simulink model "nonlinear_block"  (R2024b)
settings: Solver=ode45  StartTime=0.0  StopTime=20  FixedStep=0.01  RelTol=1e-4  AbsTol=1e-7
undefined symbols (not defined in the file): params
settings Model: Creator=david  LastModifiedBy=david

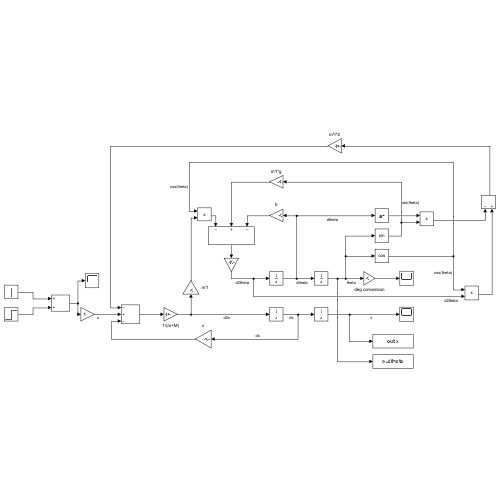
[thumbnail: Simulink's stored preview of the top-level diagram]
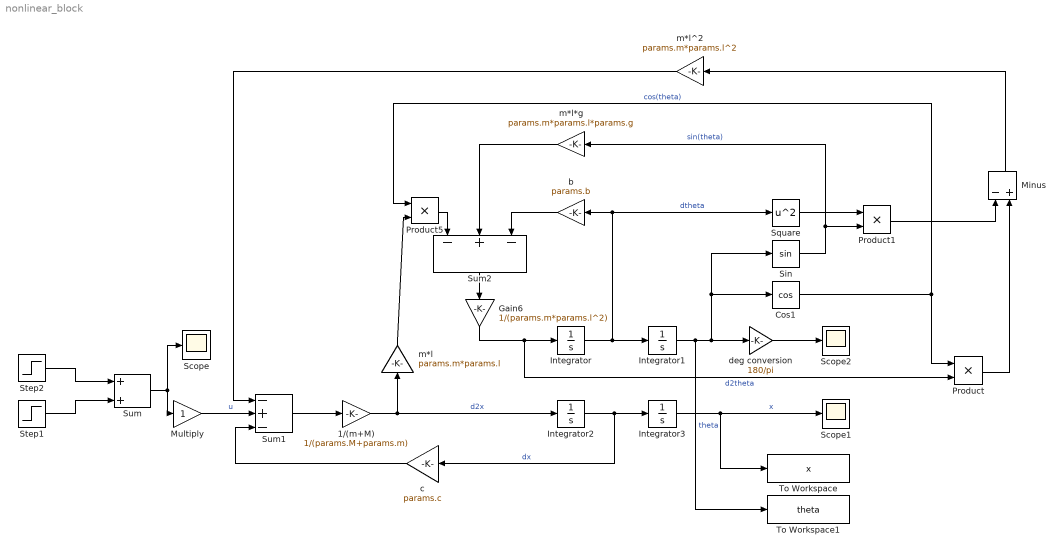
== system nonlinear_block ==
  1/(m+M) : Gain  Gain=1/(params.M+params.m)
  Cos1 : Trigonometry  Operator=cos
  Gain6 : Gain  Gain=1/(params.m*params.l^2)
  Integrator : Integrator
  Integrator1 : Integrator  InitialCondition=pi
  Integrator2 : Integrator
  Integrator3 : Integrator
  Minus : Sum  Inputs=-+
  Multiply : Gain
  Product : Product
  Product1 : Product
  Product5 : Product
  Scope : Scope
  Scope1 : Scope
  Scope2 : Scope
  Sin : Trigonometry
  Square : Math  Operator=square
  Step1 : Step  SampleTime=0
  Step2 : Step  Time=2  After=-1  SampleTime=0
  Sum : Sum
  Sum1 : Sum  Inputs=-+-
  Sum2 : Sum  Inputs=-+-
  To Workspace : ToWorkspace  VariableName=x  SampleTime=-1
      settings: Save2DSignal=2-D array (concatenate along first dimension)
  To Workspace1 : ToWorkspace  VariableName=theta  SampleTime=-1
      settings: Save2DSignal=2-D array (concatenate along first dimension)
  b : Gain  Gain=params.b
  c : Gain  Gain=params.c
  deg conversion : Gain  Gain=180/pi
  m*l : Gain  Gain=params.m*params.l
  m*l*g : Gain  Gain=params.m*params.l*params.g
  m*l^2 : Gain  Gain=params.m*params.l^2
  wires:
  Step1/1 -> Sum/2
  Step2/1 -> Sum/1
  Sum/1 -> Multiply/1, Scope/1
  Gain6/1 -> Integrator/1, Product/2  "d2theta"
  Integrator/1 -> Integrator1/1, Square/1, b/1  "dtheta"
  Integrator1/1 -> To Workspace1/1, Sin/1, Cos1/1, deg conversion/1  "theta"
  Multiply/1 -> Sum1/2  "u"
  Sum1/1 -> 1/(m+M)/1
  Product/1 -> Minus/2
  Sin/1 -> m*l*g/1, Product1/2  "sin(theta)"
  Product1/1 -> Minus/1
  Minus/1 -> m*l^2/1
  m*l^2/1 -> Sum1/1
  Integrator2/1 -> c/1, Integrator3/1  "dx"
  1/(m+M)/1 -> Integrator2/1, m*l/1  "d2x"
  Integrator3/1 -> To Workspace/1, Scope1/1  "x"
  c/1 -> Sum1/3
  Sum2/1 -> Gain6/1
  b/1 -> Sum2/3
  Product5/1 -> Sum2/1
  Cos1/1 -> Product5/1, Product/1  "cos(theta)"
  m*l*g/1 -> Sum2/2
  deg conversion/1 -> Scope2/1
  m*l/1 -> Product5/2
  Square/1 -> Product1/1
